simulink model "RTR_sim2021a"  (R2021a)
settings: Solver=ode45  StartTime=0.0  StopTime=t_stop  RelTol=1e-10
values from neighbouring files (symbols this model uses):
  g = 9.81    [RTR.m]    (also in TRT.m)
  Kd = 200    [RTR.m]
  Kp = 2000    [RTR.m]
  l2 = 0.3    [RTR.m]    (also in TRT.m)
  l3 = 0.2    [RTR.m]    (also in TRT.m)
  m2 = 20    [RTR.m]    (also in TRT.m)
  m3 = 20    [RTR.m]    (also in TRT.m)
  q1_0 = 2    [RTR.m]
  q1d_0 = 0    [RTR.m]
  q1p_0 = 0    [RTR.m]
  q2_0 = 4    [RTR.m]
  q2d_0 = 2    [RTR.m]
  q2p_0 = 0    [RTR.m]
  q3_0 = 2    [RTR.m]
  q3d_0 = 0    [RTR.m]
  q3p_0 = 0    [RTR.m]
settings Model: Creator=kacpe  LastModifiedBy=kacpe
settings DebuggingCC: UnconnectedInputMsg=none  UnconnectedOutputMsg=none  UnconnectedLineMsg=none
settings RTWCC: DLArmComputeVersion=20.02.1

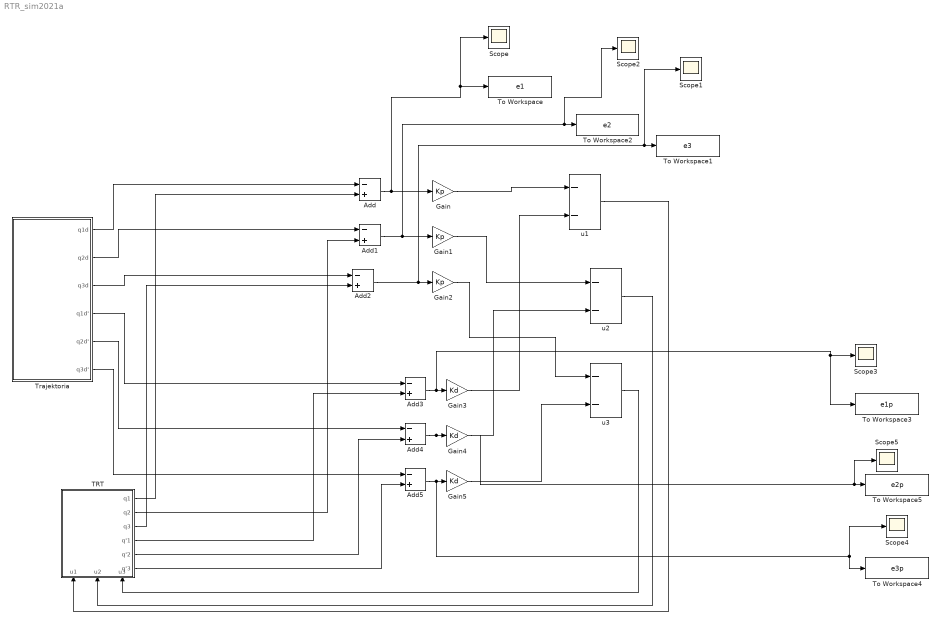
== system RTR_sim2021a ==
  Add{,1..5} (6 alike) : Sum  Inputs=-+
  Gain : Gain  Gain=Kp
  Gain1 : Gain  Gain=Kp
  Gain2 : Gain  Gain=Kp
  Gain3 : Gain  Gain=Kd
  Gain4 : Gain  Gain=Kd
  Gain5 : Gain  Gain=Kd
  Scope{,1..5} (6 alike) : Scope
  TRT : Subsystem
      settings: PortSchema="{\"entries\":[{\"content\":{\"sides\":[{\"content\":{\"connectorIds\":[]},\"type\":\"ConnectorPlacement.EquallySpacedRectSide\",\"uuid\":\"a13a475c-743e-4b68-af9c-5e746e266b9c\"},{\"content\":{\"connectorIds\":[\"Out1\",\"Out2\",\"Out3\",\"Out4\",\"Out5\",\"Out6\"],\"side\":\"RIGHT\"},\"type\":\"ConnectorPlacement.EquallySpacedRectSide\",\"uuid\":\"c38df9ec-cc79-4f7b-9920-87d5ccf64580\"},{\"content\":{\"connectorIds\":[],\"side\":\"TOP\"},\"type\":\"ConnectorPlacement.EquallySpacedRectSide\",\"uuid\":\"3e71a422-c3ba-4d07-a3dd-6a096f4f70e7\"},{\"content\":{\"connectorIds\":[\"In1\",\"In2\",\"In3\"],\"side\":\"BOTTOM\"},\"type\":\"ConnectorPlacement.EquallySpacedRectSide\",\"uuid\":\"943e58bb-edab-4cbf-b22e-e260512a1992\"}]},\"type\":\"ConnectorPlacement.EquallySpacedConnector\",\"uuid\":\"0ec18b1f-6af6-4411-842f-55149c10a846\"}],\"packageUris\":[\"http://schema.mathworks.com/mf0/Connector/R2020b\"],\"version\":\"1.0\"}"
  To Workspace : ToWorkspace  VariableName=e1  SampleTime=-1
  To Workspace1 : ToWorkspace  VariableName=e3  SampleTime=-1
  To Workspace2 : ToWorkspace  VariableName=e2  SampleTime=-1
  To Workspace3 : ToWorkspace  VariableName=e1p  SampleTime=-1
  To Workspace4 : ToWorkspace  VariableName=e3p  SampleTime=-1
  To Workspace5 : ToWorkspace  VariableName=e2p  SampleTime=-1
  Trajektoria : Subsystem
  u1 : Sum  Inputs=--
  u2 : Sum  Inputs=--
  u3 : Sum  Inputs=--
  wires:
  Trajektoria/1(q1d) -> Add/1
  Trajektoria/2(q2d) -> Add1/1
  Trajektoria/3(q3d) -> Add2/1
  Trajektoria/4(q1d') -> Add3/1
  Trajektoria/5(q2d') -> Add4/1
  Trajektoria/6(q3d') -> Add5/1
  TRT/1(q1) -> Add/2
  TRT/2(q2) -> Add1/2
  TRT/3(q3) -> Add2/2
  TRT/4(q'1) -> Add3/2
  TRT/5(q'2) -> Add4/2
  TRT/6(q'3) -> Add5/2
  Add/1 -> Gain/1, Scope/1, To Workspace/1
  Add1/1 -> Gain1/1, Scope2/1, To Workspace2/1
  Gain3/1 -> u1/2
  Gain4/1 -> u2/2
  Gain5/1 -> u3/2
  Gain/1 -> u1/1
  Gain1/1 -> u2/1
  Gain2/1 -> u3/1
  u3/1 -> TRT/3(u3)
  u2/1 -> TRT/2(u2)
  u1/1 -> TRT/1(u1)
  Add2/1 -> Scope1/1, To Workspace1/1, Gain2/1
  Add4/1 -> Scope5/1, To Workspace5/1, Gain4/1
  Add5/1 -> Scope4/1, To Workspace4/1, Gain5/1
  Add3/1 -> To Workspace3/1, Scope3/1, Gain3/1

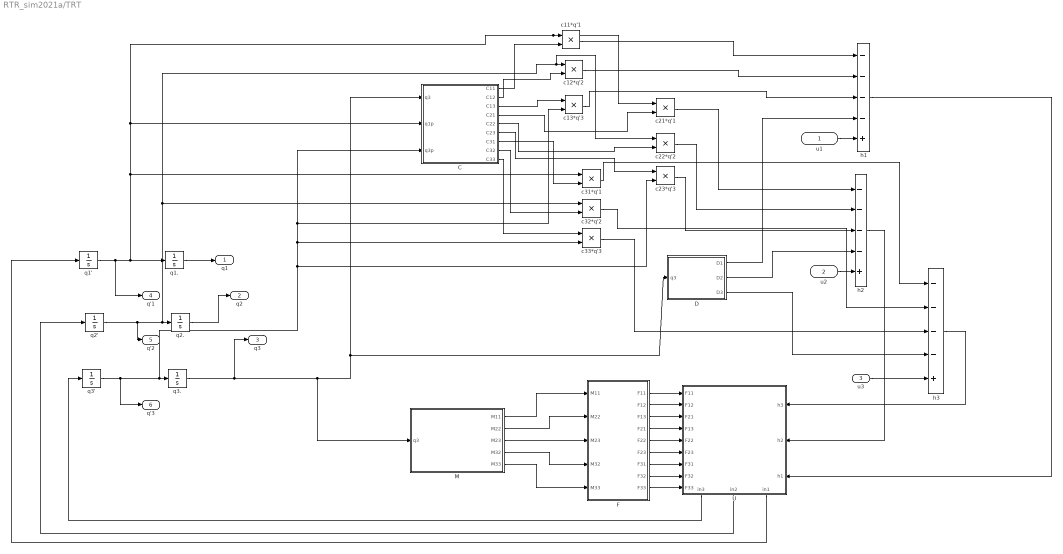
== system RTR_sim2021a/TRT ==
  u1 : Inport
  u2 : Inport  Port=2
  u3 : Inport  Port=3
  C : MATLAB Function  TreatAsAtomicUnit=on
  D : MATLAB Function  TreatAsAtomicUnit=on
  F : MATLAB Function  TreatAsAtomicUnit=on
  M : MATLAB Function  TreatAsAtomicUnit=on
  U : Subsystem
      settings: PortSchema="{\"entries\":[{\"content\":{\"sides\":[{\"content\":{\"connectorIds\":[\"In1\",\"In2\",\"In3\",\"In4\",\"In5\",\"In6\",\"In7\",\"In8\",\"In9\"]},\"type\":\"ConnectorPlacement.EquallySpacedRectSide\",\"uuid\":\"30710644-9e06-400a-91a1-da9eb46b634c\"},{\"content\":{\"connectorIds\":[\"In10\",\"In11\",\"In12\"],\"side\":\"RIGHT\"},\"type\":\"ConnectorPlacement.EquallySpacedRectSide\",\"uuid\":\"450ad47e-e867-455a-81bd-6c2cfcae7014\"},{\"content\":{\"connectorIds\":[],\"side\":\"TOP\"},\"type\":\"ConnectorPlacement.EquallySpacedRectSide\",\"uuid\":\"643bf25a-a07b-40c2-a683-349b443eb128\"},{\"content\":{\"connectorIds\":[\"Out1\",\"Out2\",\"Out3\"],\"side\":\"BOTTOM\"},\"type\":\"ConnectorPlacement.EquallySpacedRectSide\",\"uuid\":\"d7f5c48e-8c7d-4ef3-916e-98a783992e6d\"}]},\"type\":\"ConnectorPlacement.EquallySpacedConnector\",\"uuid\":\"b943515b-cd98-4c69-abf8-9cc1eb7ce306\"}],\"packageUris\":[\"http://schema.mathworks.com/mf0/Connector/R2020b\"],\"version\":\"1.0\"}"
  c11*q'1 : Product
  c12*q'2 : Product
  c13*q'3 : Product
  c21*q'1 : Product
  c22*q'2 : Product
  c23*q'3 : Product
  c31*q'1 : Product
  c32*q'2 : Product
  c33*q'3 : Product
  h1 : Sum  Inputs=----+
  h2 : Sum  Inputs=----+
  h3 : Sum  Inputs=----+
  q1' : Integrator  InitialCondition=q1p_0
  q1. : Integrator  InitialCondition=q1_0
  q2' : Integrator  InitialCondition=q2p_0
  q2. : Integrator  InitialCondition=q2_0
  q3' : Integrator  InitialCondition=q3p_0
  q3. : Integrator  InitialCondition=q3_0
  q1 : Outport
  q2 : Outport  Port=2
  q3 : Outport  Port=3
  q'1 : Outport  Port=4
  q'2 : Outport  Port=5
  q'3 : Outport  Port=6
  wires:
  M/1(M11) -> F/1(M11)
  M/2(M22) -> F/2(M22)
  M/3(M23) -> F/3(M23)
  M/4(M32) -> F/4(M32)
  M/5(M33) -> F/5(M33)
  u1/1 -> h1/5
  u3/1 -> h3/5
  u2/1 -> h2/5
  q3./1 -> C/1(q3), D/1(q3), M/1(q3), q3/1
  q3'/1 -> q'3/1, c33*q'3/2, c13*q'3/2, C/3(q3p), c23*q'3/2, q3./1
  q2'/1 -> q'2/1, c32*q'2/1, c22*q'2/1, c12*q'2/1, q2./1
  q2./1 -> q2/1
  C/1(C11) -> c11*q'1/2
  C/3(C13) -> c13*q'3/1
  C/6(C23) -> c23*q'3/1
  C/7(C31) -> c31*q'1/2
  q1./1 -> q1/1
  C/2(C12) -> c12*q'2/2
  q1'/1 -> q'1/1, c21*q'1/1, c11*q'1/1, C/2(q1p), c31*q'1/1, q1./1
  C/4(C21) -> c21*q'1/2
  C/5(C22) -> c22*q'2/2
  C/8(C32) -> c32*q'2/2
  C/9(C33) -> c33*q'3/1
  c11*q'1/1 -> h1/1
  c12*q'2/1 -> h1/2
  c13*q'3/1 -> h1/3
  D/1(D1) -> h1/4
  D/2(D2) -> h2/4
  c21*q'1/1 -> h2/1
  c22*q'2/1 -> h2/2
  D/3(D3) -> h3/4
  c31*q'1/1 -> h3/1
  c32*q'2/1 -> h3/2
  c33*q'3/1 -> h3/3
  F/1(F11) -> U/1(F11)
  F/2(F12) -> U/2(F12)
  F/3(F13) -> U/3(F21)
  F/4(F21) -> U/4(F13)
  F/5(F22) -> U/5(F22)
  F/6(F23) -> U/6(F23)
  F/7(F31) -> U/7(F31)
  F/8(F32) -> U/8(F32)
  F/9(F33) -> U/9(F33)
  h1/1 -> U/12(h1)
  h2/1 -> U/11(h2)
  h3/1 -> U/10(h3)
  U/1(in3) -> q3'/1
  U/2(in2) -> q2'/1
  U/3(in1) -> q1'/1
  c23*q'3/1 -> h2/3

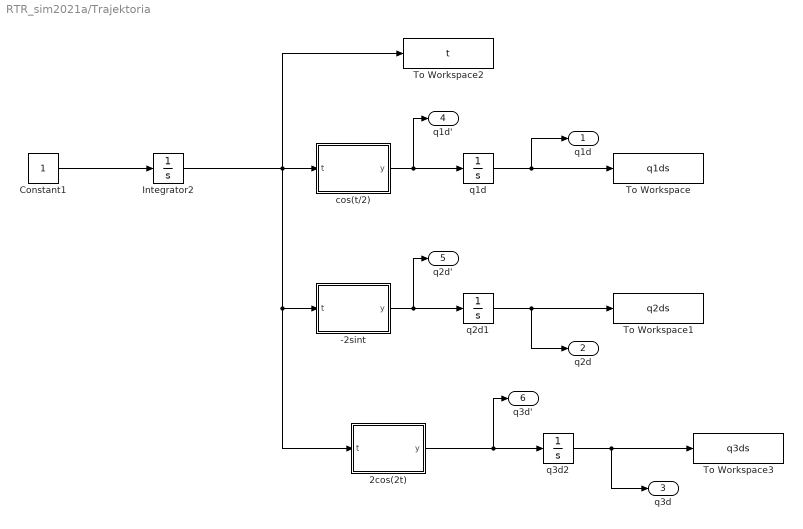
== system RTR_sim2021a/Trajektoria ==
  " q1d" : Integrator  InitialCondition=q1d_0
  " q2d1" : Integrator  InitialCondition=q2d_0
  " q3d2" : Integrator  InitialCondition=q3d_0
  -2sint : MATLAB Function  TreatAsAtomicUnit=on
  2cos(2t) : MATLAB Function  TreatAsAtomicUnit=on
  Constant1 : Constant
  Integrator2 : Integrator
  To Workspace : ToWorkspace  VariableName=q1ds  SampleTime=-1
  To Workspace1 : ToWorkspace  VariableName=q2ds  SampleTime=-1
  To Workspace2 : ToWorkspace  VariableName=t  SampleTime=-1
  To Workspace3 : ToWorkspace  VariableName=q3ds  SampleTime=-1
  cos(t/2) : MATLAB Function  TreatAsAtomicUnit=on
  q1d : Outport
  q2d : Outport  Port=2
  q3d : Outport  Port=3
  q1d' : Outport  Port=4
  q2d' : Outport  Port=5
  q3d' : Outport  Port=6
  wires:
  " q2d1"/1 -> To Workspace1/1, q2d/1
  -2sint/1(y) -> q2d'/1, " q2d1"/1
  " q1d"/1 -> To Workspace/1, q1d/1
  cos(t/2)/1(y) -> q1d'/1, " q1d"/1
  Constant1/1 -> Integrator2/1
  Integrator2/1 -> To Workspace2/1, 2cos(2t)/1(t), -2sint/1(t), cos(t/2)/1(t)
  " q3d2"/1 -> To Workspace3/1, q3d/1
  2cos(2t)/1(y) -> q3d'/1, " q3d2"/1

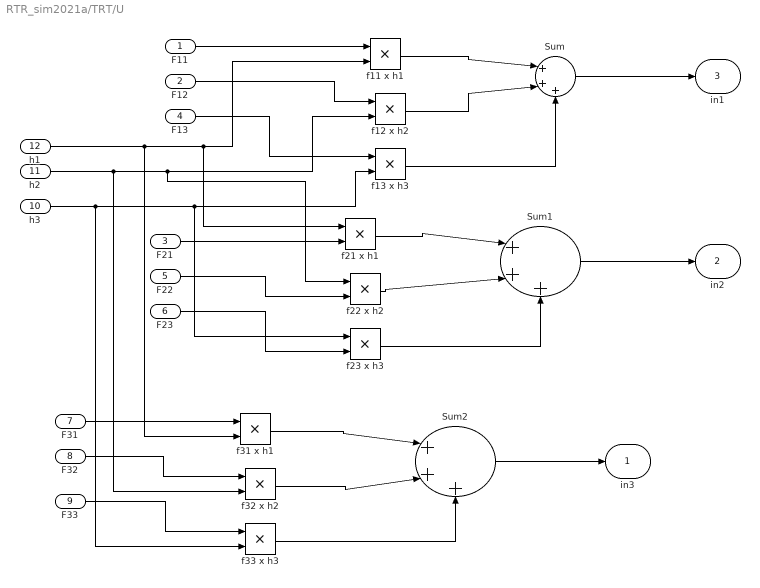
== system RTR_sim2021a/TRT/U ==
  F11 : Inport
  F12 : Inport  Port=2
  F21 : Inport  Port=3
  F13 : Inport  Port=4
  F22 : Inport  Port=5
  F23 : Inport  Port=6
  F31 : Inport  Port=7
  F32 : Inport  Port=8
  F33 : Inport  Port=9
  h3 : Inport  Port=10
  h2 : Inport  Port=11
  h1 : Inport  Port=12
  Sum : Sum  Inputs=|+++
  Sum1 : Sum  Inputs=|+++
  Sum2 : Sum  Inputs=|+++
  f11 x h1 : Product
  f12 x h2 : Product
  f13 x h3 : Product
  f21 x h1 : Product
  f22 x h2 : Product
  f23 x h3 : Product
  f31 x h1 : Product
  f32 x h2 : Product
  f33 x h3 : Product
  in3 : Outport
  in2 : Outport  Port=2
  in1 : Outport  Port=3
  wires:
  F11/1 -> f11 x h1/1
  F12/1 -> f12 x h2/1
  h2/1 -> f32 x h2/2, f22 x h2/1, f12 x h2/2
  F13/1 -> f13 x h3/1
  h3/1 -> f33 x h3/2, f23 x h3/1, f13 x h3/2
  F21/1 -> f21 x h1/2
  F22/1 -> f22 x h2/2
  F23/1 -> f23 x h3/2
  F31/1 -> f31 x h1/1
  F32/1 -> f32 x h2/1
  F33/1 -> f33 x h3/1
  h1/1 -> f31 x h1/2, f21 x h1/1, f11 x h1/2
  f11 x h1/1 -> Sum/1
  f12 x h2/1 -> Sum/2
  f13 x h3/1 -> Sum/3
  f21 x h1/1 -> Sum1/1
  f22 x h2/1 -> Sum1/2
  f23 x h3/1 -> Sum1/3
  f31 x h1/1 -> Sum2/1
  f32 x h2/1 -> Sum2/2
  f33 x h3/1 -> Sum2/3
  Sum2/1 -> in3/1
  Sum1/1 -> in2/1
  Sum/1 -> in1/1

== matlab function RTR_sim2021a/TRT/F ==
  data: M11 input; M22 input; M23 input; F11 output; M32 input; M33 input; F12 output; F13 output; F21 output; F22 output; F23 output; F31 output; F32 output; F33 output
function [F11,F12,F13,F21,F22,F23,F31,F32,F33] =fcn(M11, M22, M23, M32, M33)
%(wiersz, kolumna)
%M11, M22,  M33, M23, M32
%% output
%M=[0,0,0;0,0,0;0,0,0];
M = [M11, 0, 0;
     0, M22, M23;
     0,M32, M33];

F1 = inv(M);
F11 = F1(1,1);
F12 = F1(1,2);
F13 = F1(1,3);
F21 = F1(2,1);
F22 = F1(2,2);
F23 = F1(2,3);
F31 = F1(3,1);
F32 = F1(3,2);
F33 = F1(3,3);

== matlab function RTR_sim2021a/Trajektoria/2cos(2t) ==
  data: t input; y output
function y = fcn(t)

y = 2*cos(2*t);

== matlab function RTR_sim2021a/TRT/M ==
  data: l2 parameter; l3 parameter; m2 parameter; m3 parameter; q3 input; M11 output; M22 output; M23 output; M32 output; M33 output
function [M11, M22, M23, M32, M33] =fcn(l2,l3, m2, m3, q3)
%(wiersz, kolumna)
%M11, M22,  M33, M23, M32
%% output
%M=[0,0,0;0,0,0;0,0,0];
M11 = (1/3)*m2*(l2^2)+m3*((l2^2)+(1/3)*(l3^2)*(cos(q3)^2) + l2*l3*cos(3));
M22 = m2+m3;
M23 = (1/2)*m3*l2*l3*cos(q3);
M32 = (1/2)*m3*l2*l3*cos(q3);
M33 = (1/3)*m3*(l3^2);
%M0=0;

== matlab function RTR_sim2021a/TRT/C ==
  data: q3 input; q1p input; q3p input; m3 parameter; l2 parameter; l3 parameter; C11 output; C12 output; C13 output; C21 output; C22 output; C23 output; C31 output; C32 output; C33 output
function [C11,C12, C13,C21,C22,C23, C31,C32,C33] =fcn( q3, q1p, q3p, m3, l2, l3)
%(wiersz, kolumna)
%M11, M22,  M33, M23, M32
%% output
%M=[0,0,0;0,0,0;0,0,0];
C11 = -q3p*((1/2)*m3*l2*l3*sin(q3) + (1/3)*m3*(l3^2)*sin(q3)*cos(q3));
C13 = -q1p*((1/2)*m3*l2*l3*sin(q3) + (1/3)*m3*(l3^2)*sin(q3)*cos(q3));
C23 = -q3p*(1/2)*m3*(l3^2)*sin(q3)*cos(q3);
C31 = q1p*((1/2)*m3*l2*l3*sin(q3) + (1/3)*m3*(l3^2)*sin(q3)*cos(q3));
%C0 = 0;
C12 = 0;
C21 = 0;
C22 = 0; 
C32 = 0;
C33 = 0;

== matlab function RTR_sim2021a/TRT/D ==
  data: q3 input; m2 parameter; m3 parameter; l3 parameter; g parameter; D1 output; D2 output; D3 output
function [D1, D2, D3] =fcn(q3,m2,m3, l3, g)
%(wiersz, kolumna)
%M11, M22,  M33, M23, M32
%% output
%M=[0,0,0;0,0,0;0,0,0];
D1 = 0;
D2 = (m2+m3)*g;
D3 = (1/2)*g*m3*l3*cos(q3);

== matlab function RTR_sim2021a/Trajektoria/cos(t//2) ==
  data: t input; y output
function y = fcn(t)

y = cos(t/2);

== matlab function RTR_sim2021a/Trajektoria/-2sint ==
  data: t input; y output
function y = fcn(t)

y = -2*sin(t);
